simulink model "IMAlphaBeta"  (R2021b)
settings: Solver=VariableStepAuto  StartTime=0.0  StopTime=5  RelTol=1e-3
values from neighbouring files (symbols this model uses):
  Amp = 380    [Induction_motor_parameters.m]
  Bet = 0.068    [Induction_motor_parameters.m]
  J = [0 -1;1 0]    [Induction_motor_parameters.m]
  Jeq = 0.4    [Induction_motor_parameters.m]
  Lks_ = [Lks 0;0 Lks]    [Induction_motor_parameters.m]
  Lm_ = [Lm 0;0 Lm]    [Induction_motor_parameters.m]
  np = 3    [Induction_motor_parameters.m]
  om = 2*pi*50    (= 314.159265359)    [Induction_motor_parameters.m]
  Rr_ = [Rr 0;0 Rr]    [Induction_motor_parameters.m]
  Rs_ = [Rs 0;0 Rs]    [Induction_motor_parameters.m]
undefined symbols (not defined in the file or in its folder): Clarke, Inv_Clarke, Park
settings Model: Creator=Utente  LastModifiedBy=1
settings SolverCC: AlgebraicLoopSolver=TrustRegion
settings DataIOCC: ReturnWorkspaceOutputs=off
settings DebuggingCC: SFMachineParentedDataDiag=warning  ArithmeticOperatorsInVariantConditions=warning
settings SFSimCC: SimUseLocalCustomCode=off  CustomCodeUndefinedFunction=UseInterfaceOnly
settings RTWCC: RTWUseLocalCustomCode=off
settings CodeAppCC: StateflowObjectComments=on
settings SimscapeCC: SimscapeNormalizeSystem=off

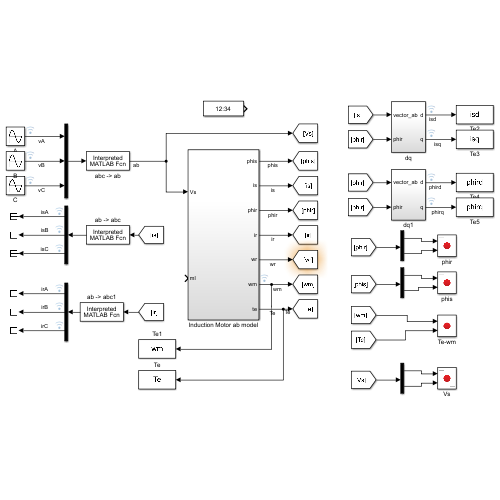
[thumbnail: Simulink's stored preview of the top-level diagram]
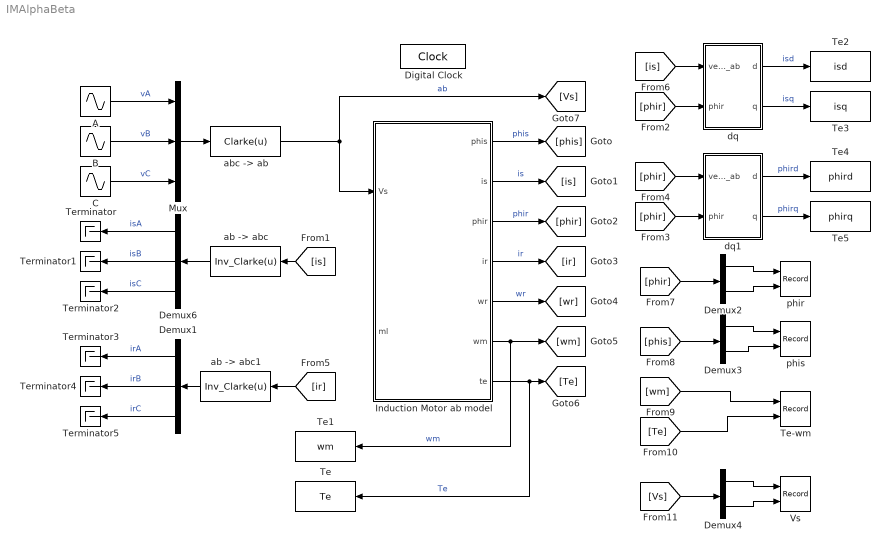
== system IMAlphaBeta ==
  A : Sin  Amplitude=Amp  Frequency=om  Phase=0 + pi/2  SampleTime=0
  B : Sin  Amplitude=Amp  Frequency=om  Phase=-2/3*pi + pi/2  SampleTime=0
  C : Sin  Amplitude=Amp  Frequency=om  Phase=2/3*pi + pi/2  SampleTime=0
  Demux1 : Demux  Outputs=3
  Demux2 : Demux  Outputs=2
  Demux3 : Demux  Outputs=2
  Demux4 : Demux  Outputs=2
  Demux6 : Demux  Outputs=3
  Digital Clock : DigitalClock  SampleTime=0.001
  Induction Motor ab model : Subsystem
  Mux : Mux  Inputs=3
  Te : ToWorkspace  VariableName=Te  SaveFormat=Timeseries  SampleTime=-1
  Te-wm : Record  FileSettingsInternal="{\"entries\":[{\"content\":{\"excelSettings\":{\"content\":{},\"type\":\"Streamout.ExcelSettings\"}},\"type\":\"Streamout.FileSettingStorage\",\"uuid\":\"bc4ad7bc-467e-46b2-91ec-95eac65564ba\"}],\"packageUris\":[\"http://schema.mathworks.com/mf0/streamout_blocks/R2020a\"],\"version\":\"1.0\"}"  Layout=[1 1]  SignalsInternal="{\"entries\":[{\"content\":{\"signals\":[{\"content\":{\"blockPath\":[\"IMAlphaBeta/Te-wm\"],\"channel\":[],\"dimensions\":[1],\"domain\":\"IMAlphaBeta/Te-wm\",\"lineColor\":\"#a2142f\",\"plots\":[1],\"port\":1,\"sid\":[\"\"],\"signalID\":2755,\"signalName\":\"From9\"},\"type\":\"RecordBlkView.Signal\",\"uuid\":\"5b3775f7-8d11-4cf7-8a02-3f1a7cbb4ad2\"},{\"content\":{\"blockPath\":[\"IMAlphaBeta/Te-wm\"],\"channel\":[],\"dimensions\":[1],\"domain\":\"IMAlphaBeta/Te-wm\",\"lineColor\":\"#139fff\",\"plots\":[1],\"port\":2,\"sid\":[\"\"],\"signalID\":2759,\"signalName\":\"From10\"},\"type\":\"RecordBlkView.Signal\",\"uuid\":\"6393f8fa-ca8d-40f3-a489-e5e4d66f54d4\"}]},\"type\":\"RecordBlkView.InputSignals\",\"uuid\":\"22714d84-138d-411e-884c-6272b14468c5\"}],\"packageUris\":[\"http://schema.mathworks.com/mf0/streamout_blocks/R2020a\"],\"version\":\"1.0\"}"  VisualizationBindings="{\"xyplotplugin\":{\"info\":[{\"series\":[{\"bindingParametersList\":[{\"parameter\":\"X-Axis\",\"signalID\":2755,\"signalName\":\"From9\"},{\"parameter\":\"Y-Axis\",\"signalID\":2759,\"signalName\":\"From10\"}],\"seriesID\":64705}],\"subplotID\":1}]}}"  CompatibilityTag=XY  st=-1
  Te1 : ToWorkspace  VariableName=wm  SaveFormat=Timeseries  SampleTime=-1
  Te2 : ToWorkspace  VariableName=isd  SaveFormat=Timeseries  SampleTime=-1
  Te3 : ToWorkspace  VariableName=isq  SaveFormat=Timeseries  SampleTime=-1
  Te4 : ToWorkspace  VariableName=phird  SaveFormat=Timeseries  SampleTime=-1
  Te5 : ToWorkspace  VariableName=phirq  SaveFormat=Timeseries  SampleTime=-1
  Terminator{,1..5} (6 alike) : Terminator
  Vs : Record  FileSettingsInternal="{\"entries\":[{\"content\":{\"excelSettings\":{\"content\":{},\"type\":\"Streamout.ExcelSettings\"}},\"type\":\"Streamout.FileSettingStorage\",\"uuid\":\"9dcb3003-91f4-4e84-9f7d-864a3e800a25\"}],\"packageUris\":[\"http://schema.mathworks.com/mf0/streamout_blocks/R2020a\"],\"version\":\"1.0\"}"  Layout=[1 1]  SignalsInternal="{\"entries\":[{\"content\":{\"signals\":[{\"content\":{\"blockPath\":[\"IMAlphaBeta/Vs\"],\"channel\":[],\"dimensions\":[1],\"domain\":\"IMAlphaBeta/Vs\",\"lineColor\":\"#a2142f\",\"plots\":[1],\"port\":1,\"sid\":[\"\"],\"signalID\":2763,\"signalName\":\"Demux4:1\"},\"type\":\"RecordBlkView.Signal\",\"uuid\":\"79428a3f-19da-4e99-9ef9-002d2b85a82d\"},{\"content\":{\"blockPath\":[\"IMAlphaBeta/Vs\"],\"channel\":[],\"dimensions\":[1],\"domain\":\"IMAlphaBeta/Vs\",\"lineColor\":\"#139fff\",\"plots\":[1],\"port\":2,\"sid\":[\"\"],\"signalID\":2767,\"signalName\":\"Demux4:2\"},\"type\":\"RecordBlkView.Signal\",\"uuid\":\"6afa77d6-0f8c-40c3-b2f4-784a1da54ef2\"}]},\"type\":\"RecordBlkView.InputSignals\",\"uuid\":\"568c4bbf-9bdf-4917-8804-6f83a76c840d\"}],\"packageUris\":[\"http://schema.mathworks.com/mf0/streamout_blocks/R2020a\"],\"version\":\"1.0\"}"  VisualizationBindings="{\"xyplotplugin\":{\"info\":[{\"series\":[{\"bindingParametersList\":[{\"parameter\":\"X-Axis\",\"signalID\":2763,\"signalName\":\"Demux4:1\"},{\"parameter\":\"Y-Axis\",\"signalID\":2767,\"signalName\":\"Demux4:2\"}],\"seriesID\":30778}],\"subplotID\":1}]}}"  CompatibilityTag=XY  st=-1
  "ab -> abc" : MATLABFcn  MATLABFcn=Inv_Clarke(u)  OutputDimensions=3
  "ab -> abc1" : MATLABFcn  MATLABFcn=Inv_Clarke(u)  OutputDimensions=3
  "abc -> ab" : MATLABFcn  MATLABFcn=Clarke(u)  OutputDimensions=2
  dq : Subsystem
  dq1 : Subsystem
  phir : Record  FileSettingsInternal="{\"entries\":[{\"content\":{\"excelSettings\":{\"content\":{},\"type\":\"Streamout.ExcelSettings\"}},\"type\":\"Streamout.FileSettingStorage\",\"uuid\":\"b957c152-4c0d-4bc4-ba22-64160a85e37f\"}],\"packageUris\":[\"http://schema.mathworks.com/mf0/streamout_blocks/R2020a\"],\"version\":\"1.0\"}"  Layout=[1 1]  SignalsInternal="{\"entries\":[{\"content\":{\"signals\":[{\"content\":{\"blockPath\":[\"IMAlphaBeta/phir\"],\"channel\":[],\"dimensions\":[1],\"domain\":\"IMAlphaBeta/phir\",\"lineColor\":\"#a2142f\",\"plots\":[1],\"port\":1,\"sid\":[\"\"],\"signalID\":2771,\"signalName\":\"Demux2:1\"},\"type\":\"RecordBlkView.Signal\",\"uuid\":\"fb801944-a432-4bb5-ae37-52e7019635a8\"},{\"content\":{\"blockPath\":[\"IMAlphaBeta/phir\"],\"channel\":[],\"dimensions\":[1],\"domain\":\"IMAlphaBeta/phir\",\"lineColor\":\"#139fff\",\"plots\":[1],\"port\":2,\"sid\":[\"\"],\"signalID\":2775,\"signalName\":\"Demux2:2\"},\"type\":\"RecordBlkView.Signal\",\"uuid\":\"16c4bfeb-10b0-441d-a6e0-2fd22489759b\"}]},\"type\":\"RecordBlkView.InputSignals\",\"uuid\":\"a4f52f70-a1cc-4838-abba-90098fb3e641\"}],\"packageUris\":[\"http://schema.mathworks.com/mf0/streamout_blocks/R2020a\"],\"version\":\"1.0\"}"  VisualizationBindings="{\"xyplotplugin\":{\"info\":[{\"series\":[{\"bindingParametersList\":[{\"parameter\":\"X-Axis\",\"signalID\":2771,\"signalName\":\"Demux2:1\"},{\"parameter\":\"Y-Axis\",\"signalID\":2775,\"signalName\":\"Demux2:2\"}],\"seriesID\":34586}],\"subplotID\":1}]}}"  CompatibilityTag=XY  st=-1
  phis : Record  FileSettingsInternal="{\"entries\":[{\"content\":{\"excelSettings\":{\"content\":{},\"type\":\"Streamout.ExcelSettings\"}},\"type\":\"Streamout.FileSettingStorage\",\"uuid\":\"e917278c-ae61-4bfc-ad42-b2daaaa60b47\"}],\"packageUris\":[\"http://schema.mathworks.com/mf0/streamout_blocks/R2020a\"],\"version\":\"1.0\"}"  Layout=[1 1]  SignalsInternal="{\"entries\":[{\"content\":{\"signals\":[{\"content\":{\"blockPath\":[\"IMAlphaBeta/phis\"],\"channel\":[],\"dimensions\":[1],\"domain\":\"IMAlphaBeta/phis\",\"lineColor\":\"#a2142f\",\"plots\":[1],\"port\":1,\"sid\":[\"\"],\"signalID\":2779,\"signalName\":\"Demux3:1\"},\"type\":\"RecordBlkView.Signal\",\"uuid\":\"d707ecb1-c22f-4e68-9267-e2aa8215428d\"},{\"content\":{\"blockPath\":[\"IMAlphaBeta/phis\"],\"channel\":[],\"dimensions\":[1],\"domain\":\"IMAlphaBeta/phis\",\"lineColor\":\"#139fff\",\"plots\":[1],\"port\":2,\"sid\":[\"\"],\"signalID\":2783,\"signalName\":\"Demux3:2\"},\"type\":\"RecordBlkView.Signal\",\"uuid\":\"0914ba62-204a-46c7-9248-6dbfe8803d3b\"}]},\"type\":\"RecordBlkView.InputSignals\",\"uuid\":\"c8351281-27cb-4961-a02a-3ed9c0008329\"}],\"packageUris\":[\"http://schema.mathworks.com/mf0/streamout_blocks/R2020a\"],\"version\":\"1.0\"}"  VisualizationBindings="{\"xyplotplugin\":{\"info\":[{\"series\":[{\"bindingParametersList\":[{\"parameter\":\"X-Axis\",\"signalID\":2779,\"signalName\":\"Demux3:1\"},{\"parameter\":\"Y-Axis\",\"signalID\":2783,\"signalName\":\"Demux3:2\"}],\"seriesID\":6872}],\"subplotID\":1}]}}"  CompatibilityTag=XY  st=-1
  wires:
  Mux/1 -> "abc -> ab"/1
  A/1 -> Mux/1  "vA"
  B/1 -> Mux/2  "vB"
  C/1 -> Mux/3  "vC"
  "abc -> ab"/1 -> [Vs], Induction Motor ab model/1(Vs)  "ab"
  "ab -> abc"/1 -> Demux6/1
  Demux6/1 -> Terminator/1  "isA"
  Demux6/2 -> Terminator1/1  "isB"
  Demux6/3 -> Terminator2/1  "isC"
  Induction Motor ab model/1(phis) -> [phis]  "phis"
  Induction Motor ab model/5(wr) -> [wr]  "wr"
  Induction Motor ab model/3(phir) -> [phir]  "phir"
  Induction Motor ab model/2(is) -> [is]  "is"
  Induction Motor ab model/4(ir) -> [ir]  "ir"
  [is] -> "ab -> abc"/1
  [phir] -> dq/2(phir)
  [is] -> dq/1(vector_ab)
  [phir] -> dq1/1(vector_ab)
  [phir] -> dq1/2(phir)
  Demux1/1 -> Terminator3/1  "irA"
  "ab -> abc1"/1 -> Demux1/1
  Demux1/2 -> Terminator4/1  "irB"
  Demux1/3 -> Terminator5/1  "irC"
  [ir] -> "ab -> abc1"/1
  dq/1(d) -> Te2/1  "isd"
  dq/2(q) -> Te3/1  "isq"
  dq1/2(q) -> Te5/1  "phirq"
  dq1/1(d) -> Te4/1  "phird"
  [phir] -> Demux2/1
  Demux2/2 -> phir/2
  Demux2/1 -> phir/1
  [phis] -> Demux3/1
  Demux3/2 -> phis/2
  Demux3/1 -> phis/1
  [wm] -> Te-wm/1
  [Te] -> Te-wm/2
  Induction Motor ab model/6(wm) -> Te1/1, [wm]  "wm"
  Induction Motor ab model/7(te) -> Te/1, [Te]  "Te"
  Demux4/1 -> Vs/1
  Demux4/2 -> Vs/2
  [Vs] -> Demux4/1

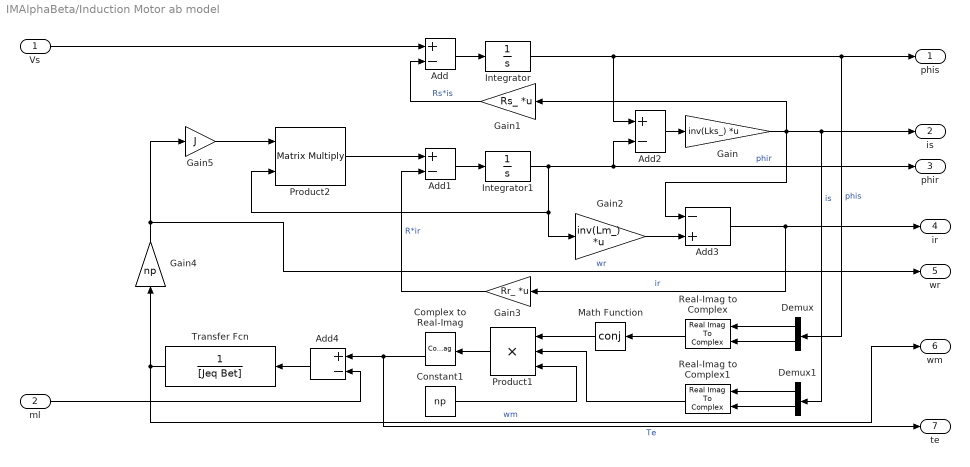
== system IMAlphaBeta/Induction Motor ab model ==
  Vs : Inport
  ml : Inport  Port=2
  Add : Sum  Inputs=+-
  Add1 : Sum  Inputs=+-  InputSameDT=on
  Add2 : Sum  Inputs=+-
  Add3 : Sum  Inputs=-+
  Add4 : Sum  Inputs=+-
  Complex to Real-Imag : ComplexToRealImag
  Constant1 : Constant  Value=np
  Demux : Demux  Outputs=2
  Demux1 : Demux  Outputs=2
  Gain : Gain  Gain=inv(Lks_)  Multiplication=Matrix(K*u)
  Gain1 : Gain  Gain=Rs_  Multiplication=Matrix(K*u)
  Gain2 : Gain  Gain=inv(Lm_)  Multiplication=Matrix(K*u)
  Gain3 : Gain  Gain=Rr_  Multiplication=Matrix(K*u)
  Gain4 : Gain  Gain=np
  Gain5 : Gain  Gain=J
  Integrator : Integrator
  Integrator1 : Integrator
  Math Function : Math  Operator=conj  SignedPower=on  SaturateOnIntegerOverflow=on
  Product1 : Product  Inputs=3
  Product2 : Product  Multiplication=Matrix(*)
  Real-Imag to Complex : RealImagToComplex
  Real-Imag to Complex1 : RealImagToComplex
  Transfer Fcn : TransferFcn  Denominator=[Jeq Bet]
  phis : Outport
  is : Outport  Port=2
  phir : Outport  Port=3
  ir : Outport  Port=4
  wr : Outport  Port=5
  wm : Outport  Port=6
  te : Outport  Port=7
  wires:
  Add1/1 -> Integrator1/1
  Gain1/1 -> Add/2  "Rs*is"
  Add/1 -> Integrator/1
  ml/1 -> Add4/2
  Constant1/1 -> Product1/3
  Add4/1 -> Transfer Fcn/1
  Complex to Real-Imag/2 -> te/1, Add4/1  "Te"
  Transfer Fcn/1 -> Gain4/1, wm/1  "wm"
  Math Function/1 -> Product1/1
  Vs/1 -> Add/1
  Product1/1 -> Complex to Real-Imag/1
  Integrator/1 -> Add2/1, Demux/1, phis/1  "phis"
  Product2/1 -> Add1/1
  Integrator1/1 -> Add2/2, phir/1, Gain2/1, Product2/2  "phir"
  Add3/1 -> ir/1, Gain3/1  "ir"
  Gain4/1 -> wr/1, Gain5/1  "wr"
  Gain/1 -> Add3/1, Demux1/1, is/1, Gain1/1  "is"
  Gain2/1 -> Add3/2
  Add2/1 -> Gain/1
  Gain3/1 -> Add1/2  "R*ir"
  Demux/2 -> Real-Imag to Complex/2
  Demux/1 -> Real-Imag to Complex/1
  Real-Imag to Complex/1 -> Math Function/1
  Demux1/2 -> Real-Imag to Complex1/2
  Demux1/1 -> Real-Imag to Complex1/1
  Real-Imag to Complex1/1 -> Product1/2
  Gain5/1 -> Product2/1

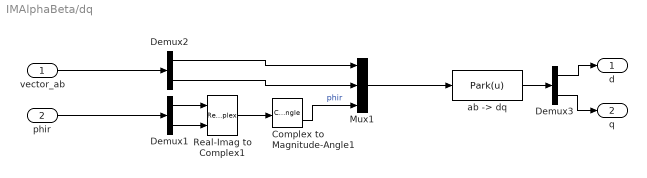
== system IMAlphaBeta/dq ==
  vector_ab : Inport
  phir : Inport  Port=2
  Complex to Magnitude-Angle1 : ComplexToMagnitudeAngle
  Demux1 : Demux  Outputs=2
  Demux2 : Demux  Outputs=2
  Demux3 : Demux  Outputs=2
  Mux1 : Mux  Inputs=3
  Real-Imag to Complex1 : RealImagToComplex
  "ab -> dq" : MATLABFcn  MATLABFcn=Park(u)
  d : Outport
  q : Outport  Port=2
  wires:
  vector_ab/1 -> Demux2/1
  Demux3/1 -> d/1
  phir/1 -> Demux1/1
  Complex to Magnitude-Angle1/2 -> Mux1/3  "phir"
  Real-Imag to Complex1/1 -> Complex to Magnitude-Angle1/1
  Demux1/2 -> Real-Imag to Complex1/2
  Demux1/1 -> Real-Imag to Complex1/1
  Demux2/1 -> Mux1/1
  Mux1/1 -> "ab -> dq"/1
  Demux2/2 -> Mux1/2
  Demux3/2 -> q/1
  "ab -> dq"/1 -> Demux3/1

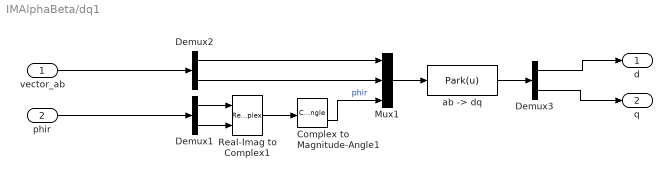
== system IMAlphaBeta/dq1 ==
  vector_ab : Inport
  phir : Inport  Port=2
  Complex to Magnitude-Angle1 : ComplexToMagnitudeAngle
  Demux1 : Demux  Outputs=2
  Demux2 : Demux  Outputs=2
  Demux3 : Demux  Outputs=2
  Mux1 : Mux  Inputs=3
  Real-Imag to Complex1 : RealImagToComplex
  "ab -> dq" : MATLABFcn  MATLABFcn=Park(u)
  d : Outport
  q : Outport  Port=2
  wires:
  vector_ab/1 -> Demux2/1
  Demux3/1 -> d/1
  phir/1 -> Demux1/1
  Complex to Magnitude-Angle1/2 -> Mux1/3  "phir"
  Real-Imag to Complex1/1 -> Complex to Magnitude-Angle1/1
  Demux1/2 -> Real-Imag to Complex1/2
  Demux1/1 -> Real-Imag to Complex1/1
  Demux2/1 -> Mux1/1
  Mux1/1 -> "ab -> dq"/1
  Demux2/2 -> Mux1/2
  Demux3/2 -> q/1
  "ab -> dq"/1 -> Demux3/1
